simulink model "ctrl_systems_3_vPID"  (Simulink 10.2)
settings: Solver=ode45  StartTime=0.0  StopTime=50  MaxStep=0.01  RelTol=1e-3  EnableMultiTasking=on
values from neighbouring files (symbols this model uses):
  A = 10    [setup_Prac5.m]
  k = k+1    (= 2)    [perf_risk.m]    (also in setup_Prac5.m = As*sqrt(2*g))
  Q = 2    [setup_Prac5.m]
  x0_ini = [2*(Q/k)^2  (Q/k)^2]    [setup_Prac5.m]
undefined symbols (not defined in the file or in its folder): Kc_zn, Td_zn, Ti_zn
settings Model: Creator=carles  LastModifiedBy=win04
settings DataIOCC: LimitDataPoints=on
settings OptimizationCC: ExpressionDepthLimit=2147483647
settings DebuggingCC: SolverPrmCheckMsg=warning  StateNameClashWarn=warning
settings ConfigComp: CovSFcnEnable=off

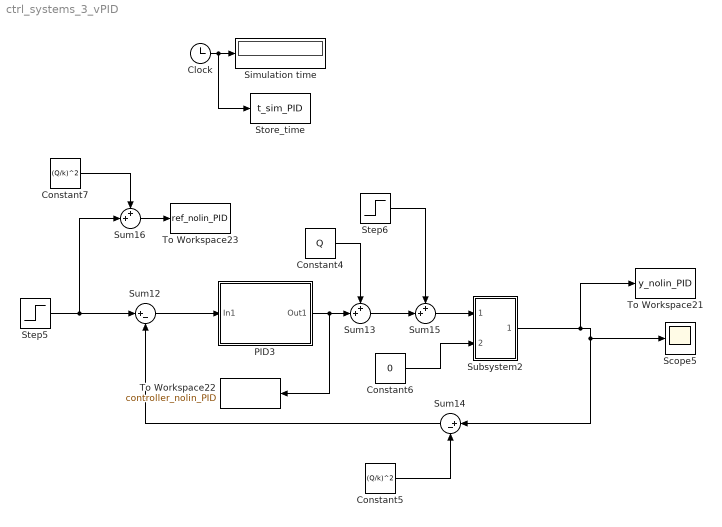
== system ctrl_systems_3_vPID ==
  Clock : Clock
  Constant4 : Constant  Value=Q
  Constant5 : Constant  Value=(Q/k)^2
  Constant6 : Constant  Value=0
  Constant7 : Constant  Value=(Q/k)^2
  PID3 : Subsystem
  Scope5 : Scope
  Simulation time : Display
  Step5 : Step  Time=10  After=0.4  SampleTime=0
  Step6 : Step  Time=30  After=0  SampleTime=0
  Store_time : ToWorkspace  VariableName=t_sim_PID
  Subsystem2 : Subsystem
  Sum12 : Sum  Inputs=|+-
  Sum13 : Sum  Inputs=++|
  Sum14 : Sum  Inputs=|+-
  Sum15 : Sum  Inputs=++|
  Sum16 : Sum  Inputs=++|
  To Workspace21 : ToWorkspace  VariableName=y_nolin_PID  SampleTime=-1
  To Workspace22 : ToWorkspace  VariableName=controller_nolin_PID  SampleTime=-1
  To Workspace23 : ToWorkspace  VariableName=ref_nolin_PID  SaveFormat=Structure With Time  SampleTime=-1
  wires:
  Sum12/1 -> PID3/1(In1)
  Subsystem2/1(Out2) -> To Workspace21/1, Sum14/1, Scope5/1
  Constant6/1 -> Subsystem2/2(In2)
  Constant4/1 -> Sum13/1
  Constant5/1 -> Sum14/2
  Sum14/1 -> Sum12/2
  PID3/1(Out1) -> To Workspace22/1, Sum13/2
  Sum15/1 -> Subsystem2/1(In1)
  Sum13/1 -> Sum15/2
  Step5/1 -> Sum16/2, Sum12/1
  Step6/1 -> Sum15/1
  Sum16/1 -> To Workspace23/1
  Constant7/1 -> Sum16/1
  Clock/1 -> Store_time/1, Simulation time/1

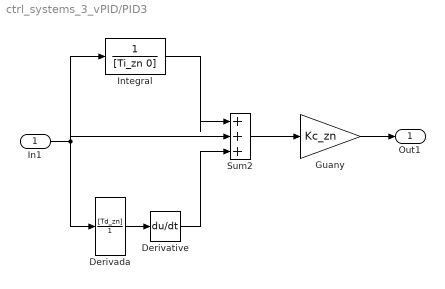
== system ctrl_systems_3_vPID/PID3 ==
  In1 : Inport
  Derivada : TransferFcn  Numerator=[Td_zn]  Denominator=[1]
  Derivative : Derivative
  Guany : Gain  Gain=Kc_zn
  Integral : TransferFcn  Denominator=[Ti_zn 0]
  Sum2 : Sum  Inputs=|+++
  Out1 : Outport
  wires:
  Derivative/1 -> Sum2/3
  Derivada/1 -> Derivative/1
  In1/1 -> Integral/1, Derivada/1, Sum2/2
  Integral/1 -> Sum2/1
  Sum2/1 -> Guany/1
  Guany/1 -> Out1/1

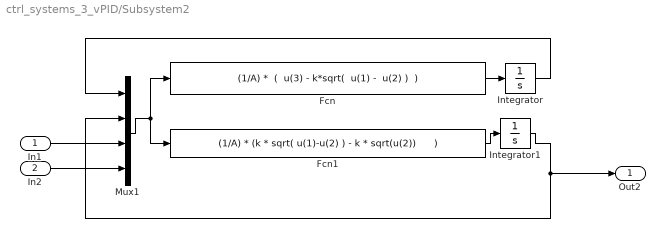
== system ctrl_systems_3_vPID/Subsystem2 ==
  In1 : Inport
  In2 : Inport  Port=2
  Fcn : Fcn  Expr="(1/A) *  (  u(3) - k*sqrt(  u(1) -  u(2) )  )"
  Fcn1 : Fcn  Expr="(1/A) * (k * sqrt( u(1)-u(2) ) - k * sqrt(u(2))      )"
  Integrator : Integrator  InitialCondition=x0_ini(1)
  Integrator1 : Integrator  InitialCondition=x0_ini(2)
  Mux1 : Mux
  Out2 : Outport
  wires:
  In1/1 -> Mux1/3
  In2/1 -> Mux1/4
  Integrator1/1 -> Out2/1, Mux1/2
  Integrator/1 -> Mux1/1
  Mux1/1 -> Fcn/1, Fcn1/1
  Fcn1/1 -> Integrator1/1
  Fcn/1 -> Integrator/1
